simulink library "Simple_lib"  (R2018b)
settings: Solver=ode45  StartTime=0.0  StopTime=10.0  RelTol=1e-3  EnableMultiTasking=on
undefined symbols (not defined in the file or in its folder): Acceptance, beta, C, C_J, C_P, c_wall, dGain, DiscIntNeverNeededParam, Duplex, Electrical_lib, grab, h_fe, i, i3, K_T, Kman, KmanCE, mu_s, n_rev, R_arm, Simplex, systemTs, tau_0, TinIC, Ts, w_0, wallMass, Watch_lib
libraries: $bdroot x407, PlantUtilityBlockset_lib x30, peGeneralControl x22, simulink x11
(part 13 of 14)

== system Simple_lib/Driveline/Changan Transmission/Synchro2/Push_out ==
  InPot : Inport
  InFlow : Inport  Tag=NOFLUX  Port=2
  OutPot : Outport  Tag=NOFLUX
  tag scope: Push_outSynchro2TransmissionHYBPTPlantHybpt_test=global
  wires:
  InPot/1 -> OutPot/1  "pot"
  InFlow/1 -> [Push_outSynchro2TransmissionHYBPTPlantHybpt_test]  "flow"

== system Simple_lib/Driveline/Changan Transmission/Synchro2/Static Friction ==
  cap : Inport
  Dw : Inport  Port=2
  w : Inport  Port=3
  Tq : Inport  Port=4
  1/R2 : Gain  Gain=mu_s/2
  Abs : Abs
  Abs1 : Abs
  Abs2 : Abs
  Delay : Delay  DelayLength=1  InitialCondition=0
  Discrete-Time Integrator : DiscreteIntegrator  gainval=k_static  ExternalReset=level  SampleTime=Ts  ICPrevOutput=DiscIntNeverNeededParam  ICPrevScaledInput=DiscIntNeverNeededParam
  Logical Operator : Logic  Operator=OR  AllPortsSameDT=off  OutDataTypeStr=boolean
  Logical Operator1 : Logic  AllPortsSameDT=off  OutDataTypeStr=boolean
  Logical Operator2 : Logic  Operator=NOT  Inputs=1  AllPortsSameDT=off  OutDataTypeStr=boolean
  Relational Operator : RelationalOperator  OutDataTypeStr=boolean  RndMeth=Nearest
  Relational Operator1 : RelationalOperator  OutDataTypeStr=boolean  RndMeth=Nearest
  Saturation1 : Saturate  UpperLimit=inf  LowerLimit=0
  Sum2 : Sum  Inputs=-++
  big speed diff : Scope
  capacity : Scope
  oldtrans_exceeds_cap : Scope
  slipping : Scope
  Tq_stat : Outport
  wires:
  1/R2/1 -> Relational Operator/2
  Relational Operator/1 -> Logical Operator/1, big speed diff/1
  cap/1 -> capacity/1, Saturation1/1
  Logical Operator/1 -> slipping/1, Discrete-Time Integrator/2
  Discrete-Time Integrator/1 -> Tq_stat/1
  Abs/1 -> Relational Operator/1
  Abs2/1 -> Relational Operator1/1
  Saturation1/1 -> Relational Operator1/2
  Abs1/1 -> 1/R2/1
  Logical Operator1/1 -> oldtrans_exceeds_cap/1, Logical Operator/2
  Sum2/1 -> Abs1/1
  Tq/1 -> Abs2/1
  w/1 -> Sum2/2, Sum2/3
  Dw/1 -> Discrete-Time Integrator/1, Abs/1, Sum2/1
  Relational Operator1/1 -> Delay/1, Logical Operator1/1
  Delay/1 -> Logical Operator2/1
  Logical Operator2/1 -> Logical Operator1/2

== system Simple_lib/Driveline/Changan Transmission/Synchro3/Dynamic Friction ==
  Dw : Inport
  cap : Inport  Port=2
  Product : Product  RndMeth=Zero
  Saturation : Saturate  UpperLimit=inf  LowerLimit=0
  friction : Trigonometry  Operator=tanh
  grab : Gain  Gain=grab
  Tq_dyn : Outport
  wires:
  Dw/1 -> grab/1
  grab/1 -> friction/1
  friction/1 -> Product/2
  cap/1 -> Saturation/1
  Saturation/1 -> Product/1
  Product/1 -> Tq_dyn/1

== system Simple_lib/Driveline/Changan Transmission/Synchro3/Push_in ==
  InPot : Inport
  InFlow : Inport  Tag=NOFLUX  Port=2
  OutPot : Outport  Tag=NOFLUX
  tag scope: Push_inSynchro3TransmissionHYBPTPlantHybpt_test=global
  wires:
  InPot/1 -> OutPot/1  "pot"
  InFlow/1 -> [Push_inSynchro3TransmissionHYBPTPlantHybpt_test]  "flow"

== system Simple_lib/Driveline/Changan Transmission/Synchro3/Push_out ==
  InPot : Inport
  InFlow : Inport  Tag=NOFLUX  Port=2
  OutPot : Outport  Tag=NOFLUX
  tag scope: Push_outSynchro3TransmissionHYBPTPlantHybpt_test=global
  wires:
  InPot/1 -> OutPot/1  "pot"
  InFlow/1 -> [Push_outSynchro3TransmissionHYBPTPlantHybpt_test]  "flow"

== system Simple_lib/Driveline/Changan Transmission/Synchro3/Static Friction ==
  cap : Inport
  Dw : Inport  Port=2
  w : Inport  Port=3
  Tq : Inport  Port=4
  1/R2 : Gain  Gain=mu_s/2
  Abs : Abs
  Abs1 : Abs
  Abs2 : Abs
  Delay : Delay  DelayLength=1  InitialCondition=0
  Discrete-Time Integrator : DiscreteIntegrator  gainval=k_static  ExternalReset=level  SampleTime=Ts  ICPrevOutput=DiscIntNeverNeededParam  ICPrevScaledInput=DiscIntNeverNeededParam
  Logical Operator : Logic  Operator=OR  AllPortsSameDT=off  OutDataTypeStr=boolean
  Logical Operator1 : Logic  AllPortsSameDT=off  OutDataTypeStr=boolean
  Logical Operator2 : Logic  Operator=NOT  Inputs=1  AllPortsSameDT=off  OutDataTypeStr=boolean
  Relational Operator : RelationalOperator  OutDataTypeStr=boolean  RndMeth=Nearest
  Relational Operator1 : RelationalOperator  OutDataTypeStr=boolean  RndMeth=Nearest
  Saturation1 : Saturate  UpperLimit=inf  LowerLimit=0
  Sum2 : Sum  Inputs=-++
  big speed diff : Scope
  capacity : Scope
  oldtrans_exceeds_cap : Scope
  slipping : Scope
  Tq_stat : Outport
  wires:
  1/R2/1 -> Relational Operator/2
  Relational Operator/1 -> Logical Operator/1, big speed diff/1
  cap/1 -> capacity/1, Saturation1/1
  Logical Operator/1 -> slipping/1, Discrete-Time Integrator/2
  Discrete-Time Integrator/1 -> Tq_stat/1
  Abs/1 -> Relational Operator/1
  Abs2/1 -> Relational Operator1/1
  Saturation1/1 -> Relational Operator1/2
  Abs1/1 -> 1/R2/1
  Logical Operator1/1 -> oldtrans_exceeds_cap/1, Logical Operator/2
  Sum2/1 -> Abs1/1
  Tq/1 -> Abs2/1
  w/1 -> Sum2/2, Sum2/3
  Dw/1 -> Discrete-Time Integrator/1, Abs/1, Sum2/1
  Relational Operator1/1 -> Delay/1, Logical Operator1/1
  Delay/1 -> Logical Operator2/1
  Logical Operator2/1 -> Logical Operator1/2

== system Simple_lib/Driveline/Changan Transmission/Synchro4/Dynamic Friction ==
  Dw : Inport
  cap : Inport  Port=2
  Product : Product  RndMeth=Zero
  Saturation : Saturate  UpperLimit=inf  LowerLimit=0
  friction : Trigonometry  Operator=tanh
  grab : Gain  Gain=grab
  Tq_dyn : Outport
  wires:
  Dw/1 -> grab/1
  grab/1 -> friction/1
  friction/1 -> Product/2
  cap/1 -> Saturation/1
  Saturation/1 -> Product/1
  Product/1 -> Tq_dyn/1

== system Simple_lib/Driveline/Changan Transmission/Synchro4/Push_in ==
  InPot : Inport
  InFlow : Inport  Tag=NOFLUX  Port=2
  OutPot : Outport  Tag=NOFLUX
  tag scope: Push_inSynchro4TransmissionHYBPTPlantHybpt_test=global
  wires:
  InPot/1 -> OutPot/1  "pot"
  InFlow/1 -> [Push_inSynchro4TransmissionHYBPTPlantHybpt_test]  "flow"

== system Simple_lib/Driveline/Changan Transmission/Synchro4/Push_out ==
  InPot : Inport
  InFlow : Inport  Tag=NOFLUX  Port=2
  OutPot : Outport  Tag=NOFLUX
  tag scope: Push_outSynchro4TransmissionHYBPTPlantHybpt_test=global
  wires:
  InPot/1 -> OutPot/1  "pot"
  InFlow/1 -> [Push_outSynchro4TransmissionHYBPTPlantHybpt_test]  "flow"

== system Simple_lib/Driveline/Changan Transmission/Synchro4/Static Friction ==
  cap : Inport
  Dw : Inport  Port=2
  w : Inport  Port=3
  Tq : Inport  Port=4
  1/R2 : Gain  Gain=mu_s/2
  Abs : Abs
  Abs1 : Abs
  Abs2 : Abs
  Delay : Delay  DelayLength=1  InitialCondition=0
  Discrete-Time Integrator : DiscreteIntegrator  gainval=k_static  ExternalReset=level  SampleTime=Ts  ICPrevOutput=DiscIntNeverNeededParam  ICPrevScaledInput=DiscIntNeverNeededParam
  Logical Operator : Logic  Operator=OR  AllPortsSameDT=off  OutDataTypeStr=boolean
  Logical Operator1 : Logic  AllPortsSameDT=off  OutDataTypeStr=boolean
  Logical Operator2 : Logic  Operator=NOT  Inputs=1  AllPortsSameDT=off  OutDataTypeStr=boolean
  Relational Operator : RelationalOperator  OutDataTypeStr=boolean  RndMeth=Nearest
  Relational Operator1 : RelationalOperator  OutDataTypeStr=boolean  RndMeth=Nearest
  Saturation1 : Saturate  UpperLimit=inf  LowerLimit=0
  Sum2 : Sum  Inputs=-++
  big speed diff : Scope
  capacity : Scope
  oldtrans_exceeds_cap : Scope
  slipping : Scope
  Tq_stat : Outport
  wires:
  1/R2/1 -> Relational Operator/2
  Relational Operator/1 -> Logical Operator/1, big speed diff/1
  cap/1 -> capacity/1, Saturation1/1
  Logical Operator/1 -> slipping/1, Discrete-Time Integrator/2
  Discrete-Time Integrator/1 -> Tq_stat/1
  Abs/1 -> Relational Operator/1
  Abs2/1 -> Relational Operator1/1
  Saturation1/1 -> Relational Operator1/2
  Abs1/1 -> 1/R2/1
  Logical Operator1/1 -> oldtrans_exceeds_cap/1, Logical Operator/2
  Sum2/1 -> Abs1/1
  Tq/1 -> Abs2/1
  w/1 -> Sum2/2, Sum2/3
  Dw/1 -> Discrete-Time Integrator/1, Abs/1, Sum2/1
  Relational Operator1/1 -> Delay/1, Logical Operator1/1
  Delay/1 -> Logical Operator2/1
  Logical Operator2/1 -> Logical Operator1/2

== system Simple_lib/Driveline/Changan Transmission/Synchro5/Dynamic Friction ==
  Dw : Inport
  cap : Inport  Port=2
  Product : Product  RndMeth=Zero
  Saturation : Saturate  UpperLimit=inf  LowerLimit=0
  friction : Trigonometry  Operator=tanh
  grab : Gain  Gain=grab
  Tq_dyn : Outport
  wires:
  Dw/1 -> grab/1
  grab/1 -> friction/1
  friction/1 -> Product/2
  cap/1 -> Saturation/1
  Saturation/1 -> Product/1
  Product/1 -> Tq_dyn/1

== system Simple_lib/Driveline/Changan Transmission/Synchro5/Push_in ==
  InPot : Inport
  InFlow : Inport  Tag=NOFLUX  Port=2
  OutPot : Outport  Tag=NOFLUX
  tag scope: Push_inSynchro5TransmissionHYBPTPlantHybpt_test=global
  wires:
  InPot/1 -> OutPot/1  "pot"
  InFlow/1 -> [Push_inSynchro5TransmissionHYBPTPlantHybpt_test]  "flow"

== system Simple_lib/Driveline/Changan Transmission/Synchro5/Push_out ==
  InPot : Inport
  InFlow : Inport  Tag=NOFLUX  Port=2
  OutPot : Outport  Tag=NOFLUX
  tag scope: Push_outSynchro5TransmissionHYBPTPlantHybpt_test=global
  wires:
  InPot/1 -> OutPot/1  "pot"
  InFlow/1 -> [Push_outSynchro5TransmissionHYBPTPlantHybpt_test]  "flow"

== system Simple_lib/Driveline/Changan Transmission/Synchro5/Static Friction ==
  cap : Inport
  Dw : Inport  Port=2
  w : Inport  Port=3
  Tq : Inport  Port=4
  1/R2 : Gain  Gain=mu_s/2
  Abs : Abs
  Abs1 : Abs
  Abs2 : Abs
  Delay : Delay  DelayLength=1  InitialCondition=0
  Discrete-Time Integrator : DiscreteIntegrator  gainval=k_static  ExternalReset=level  SampleTime=Ts  ICPrevOutput=DiscIntNeverNeededParam  ICPrevScaledInput=DiscIntNeverNeededParam
  Logical Operator : Logic  Operator=OR  AllPortsSameDT=off  OutDataTypeStr=boolean
  Logical Operator1 : Logic  AllPortsSameDT=off  OutDataTypeStr=boolean
  Logical Operator2 : Logic  Operator=NOT  Inputs=1  AllPortsSameDT=off  OutDataTypeStr=boolean
  Relational Operator : RelationalOperator  OutDataTypeStr=boolean  RndMeth=Nearest
  Relational Operator1 : RelationalOperator  OutDataTypeStr=boolean  RndMeth=Nearest
  Saturation1 : Saturate  UpperLimit=inf  LowerLimit=0
  Sum2 : Sum  Inputs=-++
  big speed diff : Scope
  capacity : Scope
  oldtrans_exceeds_cap : Scope
  slipping : Scope
  Tq_stat : Outport
  wires:
  1/R2/1 -> Relational Operator/2
  Relational Operator/1 -> Logical Operator/1, big speed diff/1
  cap/1 -> capacity/1, Saturation1/1
  Logical Operator/1 -> slipping/1, Discrete-Time Integrator/2
  Discrete-Time Integrator/1 -> Tq_stat/1
  Abs/1 -> Relational Operator/1
  Abs2/1 -> Relational Operator1/1
  Saturation1/1 -> Relational Operator1/2
  Abs1/1 -> 1/R2/1
  Logical Operator1/1 -> oldtrans_exceeds_cap/1, Logical Operator/2
  Sum2/1 -> Abs1/1
  Tq/1 -> Abs2/1
  w/1 -> Sum2/2, Sum2/3
  Dw/1 -> Discrete-Time Integrator/1, Abs/1, Sum2/1
  Relational Operator1/1 -> Delay/1, Logical Operator1/1
  Delay/1 -> Logical Operator2/1
  Logical Operator2/1 -> Logical Operator1/2

== system Simple_lib/Driveline/Changan Transmission/Synchro6/Dynamic Friction ==
  Dw : Inport
  cap : Inport  Port=2
  Product : Product  RndMeth=Zero
  Saturation : Saturate  UpperLimit=inf  LowerLimit=0
  friction : Trigonometry  Operator=tanh
  grab : Gain  Gain=grab
  Tq_dyn : Outport
  wires:
  Dw/1 -> grab/1
  grab/1 -> friction/1
  friction/1 -> Product/2
  cap/1 -> Saturation/1
  Saturation/1 -> Product/1
  Product/1 -> Tq_dyn/1

== system Simple_lib/Driveline/Changan Transmission/Synchro6/Push_in ==
  InPot : Inport
  InFlow : Inport  Tag=NOFLUX  Port=2
  OutPot : Outport  Tag=NOFLUX
  tag scope: Push_inSynchro6TransmissionHYBPTPlantHybpt_test=global
  wires:
  InPot/1 -> OutPot/1  "pot"
  InFlow/1 -> [Push_inSynchro6TransmissionHYBPTPlantHybpt_test]  "flow"

== system Simple_lib/Driveline/Changan Transmission/Synchro6/Push_out ==
  InPot : Inport
  InFlow : Inport  Tag=NOFLUX  Port=2
  OutPot : Outport  Tag=NOFLUX
  tag scope: Push_outSynchro6TransmissionHYBPTPlantHybpt_test=global
  wires:
  InPot/1 -> OutPot/1  "pot"
  InFlow/1 -> [Push_outSynchro6TransmissionHYBPTPlantHybpt_test]  "flow"

== system Simple_lib/Driveline/Changan Transmission/Synchro6/Static Friction ==
  cap : Inport
  Dw : Inport  Port=2
  w : Inport  Port=3
  Tq : Inport  Port=4
  1/R2 : Gain  Gain=mu_s/2
  Abs : Abs
  Abs1 : Abs
  Abs2 : Abs
  Delay : Delay  DelayLength=1  InitialCondition=0
  Discrete-Time Integrator : DiscreteIntegrator  gainval=k_static  ExternalReset=level  SampleTime=Ts  ICPrevOutput=DiscIntNeverNeededParam  ICPrevScaledInput=DiscIntNeverNeededParam
  Logical Operator : Logic  Operator=OR  AllPortsSameDT=off  OutDataTypeStr=boolean
  Logical Operator1 : Logic  AllPortsSameDT=off  OutDataTypeStr=boolean
  Logical Operator2 : Logic  Operator=NOT  Inputs=1  AllPortsSameDT=off  OutDataTypeStr=boolean
  Relational Operator : RelationalOperator  OutDataTypeStr=boolean  RndMeth=Nearest
  Relational Operator1 : RelationalOperator  OutDataTypeStr=boolean  RndMeth=Nearest
  Saturation1 : Saturate  UpperLimit=inf  LowerLimit=0
  Sum2 : Sum  Inputs=-++
  big speed diff : Scope
  capacity : Scope
  oldtrans_exceeds_cap : Scope
  slipping : Scope
  Tq_stat : Outport
  wires:
  1/R2/1 -> Relational Operator/2
  Relational Operator/1 -> Logical Operator/1, big speed diff/1
  cap/1 -> capacity/1, Saturation1/1
  Logical Operator/1 -> slipping/1, Discrete-Time Integrator/2
  Discrete-Time Integrator/1 -> Tq_stat/1
  Abs/1 -> Relational Operator/1
  Abs2/1 -> Relational Operator1/1
  Saturation1/1 -> Relational Operator1/2
  Abs1/1 -> 1/R2/1
  Logical Operator1/1 -> oldtrans_exceeds_cap/1, Logical Operator/2
  Sum2/1 -> Abs1/1
  Tq/1 -> Abs2/1
  w/1 -> Sum2/2, Sum2/3
  Dw/1 -> Discrete-Time Integrator/1, Abs/1, Sum2/1
  Relational Operator1/1 -> Delay/1, Logical Operator1/1
  Delay/1 -> Logical Operator2/1
  Logical Operator2/1 -> Logical Operator1/2

== system Simple_lib/Driveline/diff_R/Carrier/Duplex ==
  InPot : Inport  Tag=NOFLUX
  FlowGain : Gain
  FlowSum : Sum  Inputs=2  SaturateOnIntegerOverflow=on  InputSameDT=on  OutDataTypeStr=Inherit: Same as first input
  OutPot : Outport
  OutFlow : Outport  Tag=NOFLUX  Port=2
  wires:
  FlowGain/1 -> OutFlow/1  "out_DuplexCarrierdiff_RBEVPlantBEV"
  InPot/1 -> OutPot/1  "DuplexCarrierdiff_RBEVPlantBEV"
  FlowSum/1 -> FlowGain/1
  [SimplexTransducerERADBEVPlantBEV] -> FlowSum/1
  [PushInertiaERADBEVPlantBEV] -> FlowSum/2

== system Simple_lib/Driveline/diff_R/Carrier/Simplex ==
  InPot : Inport
  InFlow : Inport  Tag=NOFLUX  Port=2
  OutPot : Outport  Tag=NOFLUX
  tag scope: SimplexCarrierdiff_RBEVPlantBEV=global
  wires:
  InPot/1 -> OutPot/1  "SimplexCarrierdiff_RBEVPlantBEV"
  InFlow/1 -> [SimplexCarrierdiff_RBEVPlantBEV]  "out_SimplexCarrierdiff_RBEVPlantBEV"

== system Simple_lib/Driveline/diff_R/Carrier/Simplex1 ==
  InPot : Inport
  InFlow : Inport  Tag=NOFLUX  Port=2
  OutPot : Outport  Tag=NOFLUX
  tag scope: Simplex1Carrierdiff_RBEVPlantBEV=global
  wires:
  InPot/1 -> OutPot/1  "Simplex1Carrierdiff_RBEVPlantBEV"
  InFlow/1 -> [Simplex1Carrierdiff_RBEVPlantBEV]  "out_Simplex1Carrierdiff_RBEVPlantBEV"

== system Simple_lib/Driveline/diff_R/GearPair /Pull ==
  InPot : Inport  Tag=NOFLUX
  FlowGain : Gain
  OutPot : Outport
  OutFlow : Outport  Tag=NOFLUX  Port=2
  wires:
  FlowGain/1 -> OutFlow/1  "out_PullGearPairdiff_RBEVPlantBEV"
  InPot/1 -> OutPot/1  "PullGearPairdiff_RBEVPlantBEV"
  [SimplexCarrierdiff_RBEVPlantBEV] -> FlowGain/1

== system Simple_lib/Driveline/diff_R/GearPair /Push ==
  InPot : Inport
  InFlow : Inport  Tag=NOFLUX  Port=2
  OutPot : Outport  Tag=NOFLUX
  tag scope: PushGearPairdiff_RBEVPlantBEV=global
  wires:
  InPot/1 -> OutPot/1  "PushGearPairdiff_RBEVPlantBEV"
  InFlow/1 -> [PushGearPairdiff_RBEVPlantBEV]  "out_PushGearPairdiff_RBEVPlantBEV"

== system Simple_lib/Driveline/diff_R/GearPair 1/Pull ==
  InPot : Inport  Tag=NOFLUX
  FlowGain : Gain
  OutPot : Outport
  OutFlow : Outport  Tag=NOFLUX  Port=2
  wires:
  FlowGain/1 -> OutFlow/1  "out_PullGearPair1diff_RBEVPlantBEV"
  InPot/1 -> OutPot/1  "PullGearPair1diff_RBEVPlantBEV"
  [Simplex1Carrierdiff_RBEVPlantBEV] -> FlowGain/1

== system Simple_lib/Driveline/diff_R/GearPair 1/Push ==
  InPot : Inport
  InFlow : Inport  Tag=NOFLUX  Port=2
  OutPot : Outport  Tag=NOFLUX
  tag scope: PushGearPair1diff_RBEVPlantBEV=global
  wires:
  InPot/1 -> OutPot/1  "PushGearPair1diff_RBEVPlantBEV"
  InFlow/1 -> [PushGearPair1diff_RBEVPlantBEV]  "out_PushGearPair1diff_RBEVPlantBEV"

== system Simple_lib/Electrical/B2/C/Duplex ==
  potential : Inport  Tag=NOFLUX
  Display1 : Display
  duplexFluxSum : Sum  Inputs=2  SaturateOnIntegerOverflow=on  InputSameDT=on  OutDataTypeStr=Inherit: Same as first input
  fDuplexR1Duplicity1 : Scope
  pDuplexR1Duplicity1 : Scope
  potDisplay : Display
  duplex : Outport
  flow : Outport  Tag=NOFLUX  Port=2
  wires:
  potential/1 -> pDuplexR1Duplicity1/1, potDisplay/1, duplex/1
  duplexFluxSum/1 -> Display1/1, fDuplexR1Duplicity1/1, flow/1
  [duplexSimplexR0B1Duplicity1] -> duplexFluxSum/1
  [duplexSimplex1LB1Duplicity1] -> duplexFluxSum/2

== system Simple_lib/Electrical/B2/E/Duplex ==
  potential : Inport  Tag=NOFLUX
  Display1 : Display
  duplexFluxSum : Gain  SaturateOnIntegerOverflow=on  OutDataTypeStr=Inherit: Same as input  ParamDataTypeStr=Inherit: Same as input
  fDuplexR1Duplicity1 : Scope
  pDuplexR1Duplicity1 : Scope
  potDisplay : Display
  duplex : Outport
  flow : Outport  Tag=NOFLUX  Port=2
  wires:
  potential/1 -> pDuplexR1Duplicity1/1, potDisplay/1, duplex/1
  duplexFluxSum/1 -> Display1/1, fDuplexR1Duplicity1/1, flow/1
  [duplexSimplexLB1Duplicity1] -> duplexFluxSum/1

== system Simple_lib/Electrical/B2/E/Simplex ==
  duplex : Inport
  In2 : Inport  Tag=NOFLUX  Port=2
  fSimplexR1Duplicity1 : Scope
  flowDisplay : Display
  fluxduplexGain : Gain  SaturateOnIntegerOverflow=on  OutDataTypeStr=Inherit: Same as input  ParamDataTypeStr=Inherit: Same as input
  pSimplexR1Duplicity1 : Scope
  potDisplay : Display
  simplex : Outport  Tag=NOFLUX
  tag scope: duplexSimplexEB1Duplicity1=global
  wires:
  In2/1 -> fSimplexR1Duplicity1/1, fluxduplexGain/1, flowDisplay/1
  fluxduplexGain/1 -> [duplexSimplexEB1Duplicity1]
  duplex/1 -> potDisplay/1, pSimplexR1Duplicity1/1, simplex/1

== system Simple_lib/Electrical/B2/L/Simplex ==
  duplex : Inport
  In2 : Inport  Tag=NOFLUX  Port=2
  fSimplexR1Duplicity1 : Scope
  flowDisplay : Display
  fluxduplexGain : Gain  SaturateOnIntegerOverflow=on  OutDataTypeStr=Inherit: Same as input  ParamDataTypeStr=Inherit: Same as input
  pSimplexR1Duplicity1 : Scope
  potDisplay : Display
  simplex : Outport  Tag=NOFLUX
  tag scope: duplexSimplexLB1Duplicity1=global
  wires:
  In2/1 -> fSimplexR1Duplicity1/1, fluxduplexGain/1, flowDisplay/1
  fluxduplexGain/1 -> [duplexSimplexLB1Duplicity1]
  duplex/1 -> potDisplay/1, pSimplexR1Duplicity1/1, simplex/1

== system Simple_lib/Electrical/B2/L/Simplex1 ==
  duplex : Inport
  In2 : Inport  Tag=NOFLUX  Port=2
  fSimplexR1Duplicity1Simplex1LB1Duplicity1 : Scope
  flowDisplay : Display
  fluxduplexGain : Gain  SaturateOnIntegerOverflow=on  OutDataTypeStr=Inherit: Same as input  ParamDataTypeStr=Inherit: Same as input
  pSimplexR1Duplicity1Simplex1LB1Duplicity1 : Scope
  potDisplay : Display
  simplex : Outport  Tag=NOFLUX
  tag scope: duplexSimplex1LB1Duplicity1=global
  wires:
  In2/1 -> fSimplexR1Duplicity1Simplex1LB1Duplicity1/1, fluxduplexGain/1, flowDisplay/1
  fluxduplexGain/1 -> [duplexSimplex1LB1Duplicity1]
  duplex/1 -> potDisplay/1, pSimplexR1Duplicity1Simplex1LB1Duplicity1/1, simplex/1

== system Simple_lib/Electrical/B2/R0/Duplex ==
  potential : Inport  Tag=NOFLUX
  Display1 : Display
  duplexFluxSum : Gain  SaturateOnIntegerOverflow=on  OutDataTypeStr=Inherit: Same as input  ParamDataTypeStr=Inherit: Same as input
  fDuplexR1Duplicity1 : Scope
  pDuplexR1Duplicity1 : Scope
  potDisplay : Display
  duplex : Outport
  flow : Outport  Tag=NOFLUX  Port=2
  wires:
  potential/1 -> pDuplexR1Duplicity1/1, potDisplay/1, duplex/1
  duplexFluxSum/1 -> Display1/1, fDuplexR1Duplicity1/1, flow/1
  [duplexSimplexR1Duplicity1] -> duplexFluxSum/1

== system Simple_lib/Electrical/B2/R0/Simplex ==
  duplex : Inport
  In2 : Inport  Tag=NOFLUX  Port=2
  fSimplexR1Duplicity1 : Scope
  flowDisplay : Display
  fluxduplexGain : Gain  SaturateOnIntegerOverflow=on  OutDataTypeStr=Inherit: Same as input  ParamDataTypeStr=Inherit: Same as input
  pSimplexR1Duplicity1 : Scope
  potDisplay : Display
  simplex : Outport  Tag=NOFLUX
  tag scope: duplexSimplexR0B1Duplicity1=global
  wires:
  In2/1 -> fSimplexR1Duplicity1/1, fluxduplexGain/1, flowDisplay/1
  fluxduplexGain/1 -> [duplexSimplexR0B1Duplicity1]
  duplex/1 -> potDisplay/1, pSimplexR1Duplicity1/1, simplex/1

== system Simple_lib/Electrical/SimplestEMachine/Inertia/Push ==
  InPot : Inport
  InFlow : Inport  Tag=NOFLUX  Port=2
  OutPot : Outport  Tag=NOFLUX
  tag scope: PushInertiaEFADBEVPlantBEV=global
  wires:
  InPot/1 -> OutPot/1  "PushInertiaEFADBEVPlantBEV"
  InFlow/1 -> [PushInertiaEFADBEVPlantBEV]  "out_PushInertiaEFADBEVPlantBEV"

== system Simple_lib/Electrical/SimplestEMachine/Transducer/Duplex ==
  InPot : Inport  Tag=NOFLUX
  FlowGain : Gain
  OutPot : Outport
  OutFlow : Outport  Tag=NOFLUX  Port=2
  wires:
  [SimplexInverter_FBEVPlantBEV] -> FlowGain/1
  InPot/1 -> OutPot/1  "DuplexTransducerEFADBEVPlantBEV"
  FlowGain/1 -> OutFlow/1  "out_DuplexTransducerEFADBEVPlantBEV"

== system Simple_lib/Electrical/SimplestEMachine/Transducer/Simplex ==
  InPot : Inport
  InFlow : Inport  Tag=NOFLUX  Port=2
  OutPot : Outport  Tag=NOFLUX
  tag scope: SimplexTransducerEFADBEVPlantBEV=global
  wires:
  InFlow/1 -> [SimplexTransducerEFADBEVPlantBEV]  "out_SimplexTransducerEFADBEVPlantBEV"
  InPot/1 -> OutPot/1  "SimplexTransducerEFADBEVPlantBEV"

== system Simple_lib/Electrical/Windings/IM/Duplex ==
  InPot : Inport  Tag=NOFLUX
  FlowDisplay : Display
  FlowGain : Gain
  Flow_DuplexIMWindingsMk4v3Inverter_test0 : Scope
      settings: Tag=Flow
  PotDisplay : Display
  Pot_DuplexIMWindingsMk4v3Inverter_test0 : Scope
      settings: Tag=Pot
  Rate Transition : RateTransition  OutPortSampleTimeMultiple=nT  OutPortSampleTime=Ts
  OutPot : Outport
  OutFlow : Outport  Tag=NOFLUX  Port=2
  wires:
  Rate Transition/1 -> OutPot/1
  InPot/1 -> Rate Transition/1, PotDisplay/1, Pot_DuplexIMWindingsMk4v3Inverter_test0/1
  FlowGain/1 -> OutFlow/1, FlowDisplay/1, Flow_DuplexIMWindingsMk4v3Inverter_test0/1
  [SimplexL1WindingsMk4v3Inverter_test0] -> FlowGain/1

== system Simple_lib/Electrical/Windings/IM/Simplex ==
  InPot : Inport
  InFlow : Inport  Tag=NOFLUX  Port=2
  FlowDisplay : Display
  Flow_SimplexIMWindingsMk4v3Inverter_test0 : Scope
      settings: Tag=Flow
  PotDisplay : Display
  Pot_SimplexIMWindingsMk4v3Inverter_test0 : Scope
      settings: Tag=Pot
  Rate Transition : RateTransition  OutPortSampleTimeMultiple=Ts  OutPortSampleTime=Ts
  OutPot : Outport  Tag=NOFLUX
  tag scope: SimplexIMWindingsMk4v3Inverter_test0=global
  wires:
  InPot/1 -> Rate Transition/1
  InFlow/1 -> Flow_SimplexIMWindingsMk4v3Inverter_test0/1, FlowDisplay/1, [SimplexIMWindingsMk4v3Inverter_test0]
  Rate Transition/1 -> OutPot/1, Pot_SimplexIMWindingsMk4v3Inverter_test0/1, PotDisplay/1

== system Simple_lib/Electrical/Windings/IM1/Duplex ==
  InPot : Inport  Tag=NOFLUX
  FlowDisplay : Display
  FlowGain : Gain
  Flow_DuplexIM1WindingsMk4v3Inverter_test0 : Scope
      settings: Tag=Flow
  PotDisplay : Display
  Pot_DuplexIM1WindingsMk4v3Inverter_test0 : Scope
      settings: Tag=Pot
  Rate Transition : RateTransition  OutPortSampleTimeMultiple=nT  OutPortSampleTime=Ts
  OutPot : Outport
  OutFlow : Outport  Tag=NOFLUX  Port=2
  wires:
  Rate Transition/1 -> OutPot/1
  InPot/1 -> Rate Transition/1, PotDisplay/1, Pot_DuplexIM1WindingsMk4v3Inverter_test0/1
  FlowGain/1 -> OutFlow/1, Flow_DuplexIM1WindingsMk4v3Inverter_test0/1, FlowDisplay/1
  [SimplexL2WindingsMk4v3Inverter_test0] -> FlowGain/1

== system Simple_lib/Electrical/Windings/IM1/Simplex ==
  InPot : Inport
  InFlow : Inport  Tag=NOFLUX  Port=2
  FlowDisplay : Display
  Flow_SimplexIM1WindingsMk4v3Inverter_test0 : Scope
      settings: Tag=Flow
  PotDisplay : Display
  Pot_SimplexIM1WindingsMk4v3Inverter_test0 : Scope
      settings: Tag=Pot
  Rate Transition : RateTransition  OutPortSampleTimeMultiple=Ts  OutPortSampleTime=Ts
  OutPot : Outport  Tag=NOFLUX
  tag scope: SimplexIM1WindingsMk4v3Inverter_test0=global
  wires:
  InPot/1 -> Rate Transition/1
  InFlow/1 -> Flow_SimplexIM1WindingsMk4v3Inverter_test0/1, FlowDisplay/1, [SimplexIM1WindingsMk4v3Inverter_test0]
  Rate Transition/1 -> OutPot/1, Pot_SimplexIM1WindingsMk4v3Inverter_test0/1, PotDisplay/1

== system Simple_lib/Electrical/Windings/IM2/Duplex ==
  InPot : Inport  Tag=NOFLUX
  FlowDisplay : Display
  FlowGain : Gain
  Flow_DuplexIM2WindingsMk4v3Inverter_test0 : Scope
      settings: Tag=Flow
  PotDisplay : Display
  Pot_DuplexIM2WindingsMk4v3Inverter_test0 : Scope
      settings: Tag=Pot
  Rate Transition : RateTransition  OutPortSampleTimeMultiple=nT  OutPortSampleTime=Ts
  OutPot : Outport
  OutFlow : Outport  Tag=NOFLUX  Port=2
  wires:
  Rate Transition/1 -> OutPot/1
  InPot/1 -> Rate Transition/1, PotDisplay/1, Pot_DuplexIM2WindingsMk4v3Inverter_test0/1
  FlowGain/1 -> OutFlow/1, Flow_DuplexIM2WindingsMk4v3Inverter_test0/1, FlowDisplay/1
  [SimplexL3WindingsMk4v3Inverter_test0] -> FlowGain/1

== system Simple_lib/Electrical/Windings/IM2/Simplex ==
  InPot : Inport
  InFlow : Inport  Tag=NOFLUX  Port=2
  FlowDisplay : Display
  Flow_SimplexIM2WindingsMk4v3Inverter_test0 : Scope
      settings: Tag=Flow
  PotDisplay : Display
  Pot_SimplexIM2WindingsMk4v3Inverter_test0 : Scope
      settings: Tag=Pot
  Rate Transition : RateTransition  OutPortSampleTimeMultiple=Ts  OutPortSampleTime=Ts
  OutPot : Outport  Tag=NOFLUX
  tag scope: SimplexIM2WindingsMk4v3Inverter_test0=global
  wires:
  InPot/1 -> Rate Transition/1
  InFlow/1 -> Flow_SimplexIM2WindingsMk4v3Inverter_test0/1, FlowDisplay/1, [SimplexIM2WindingsMk4v3Inverter_test0]
  Rate Transition/1 -> OutPot/1, Pot_SimplexIM2WindingsMk4v3Inverter_test0/1, PotDisplay/1

== system Simple_lib/Electrical/Windings/L1/Simplex ==
  InPot : Inport
  InFlow : Inport  Tag=NOFLUX  Port=2
  FlowDisplay : Display
  Flow_SimplexL1WindingsMk4v3Inverter_test0 : Scope
      settings: Tag=Flow
  PotDisplay : Display
  Pot_SimplexL1WindingsMk4v3Inverter_test0 : Scope
      settings: Tag=Pot
  Rate Transition : RateTransition  OutPortSampleTimeMultiple=Ts  OutPortSampleTime=Ts
  OutPot : Outport  Tag=NOFLUX
  tag scope: SimplexL1WindingsMk4v3Inverter_test0=global
  wires:
  InPot/1 -> Rate Transition/1
  InFlow/1 -> Flow_SimplexL1WindingsMk4v3Inverter_test0/1, FlowDisplay/1, [SimplexL1WindingsMk4v3Inverter_test0]
  Rate Transition/1 -> OutPot/1, Pot_SimplexL1WindingsMk4v3Inverter_test0/1, PotDisplay/1

== system Simple_lib/Electrical/Windings/L1/Simplex1 ==
  InPot : Inport
  InFlow : Inport  Tag=NOFLUX  Port=2
  FlowDisplay : Display
  Flow_Simplex1L1WindingsMk4v3Inverter_test0 : Scope
      settings: Tag=Flow
  PotDisplay : Display
  Pot_Simplex1L1WindingsMk4v3Inverter_test0 : Scope
      settings: Tag=Pot
  Rate Transition : RateTransition  OutPortSampleTimeMultiple=Ts  OutPortSampleTime=Ts
  OutPot : Outport  Tag=NOFLUX
  tag scope: Simplex1L1WindingsMk4v3Inverter_test0=global
  wires:
  InPot/1 -> Rate Transition/1
  InFlow/1 -> Flow_Simplex1L1WindingsMk4v3Inverter_test0/1, FlowDisplay/1, [Simplex1L1WindingsMk4v3Inverter_test0]
  Rate Transition/1 -> OutPot/1, Pot_Simplex1L1WindingsMk4v3Inverter_test0/1, PotDisplay/1

== system Simple_lib/Electrical/Windings/L2/Simplex ==
  InPot : Inport
  InFlow : Inport  Tag=NOFLUX  Port=2
  FlowDisplay : Display
  Flow_SimplexL2WindingsMk4v3Inverter_test0 : Scope
      settings: Tag=Flow
  PotDisplay : Display
  Pot_SimplexL2WindingsMk4v3Inverter_test0 : Scope
      settings: Tag=Pot
  Rate Transition : RateTransition  OutPortSampleTimeMultiple=Ts  OutPortSampleTime=Ts
  OutPot : Outport  Tag=NOFLUX
  tag scope: SimplexL2WindingsMk4v3Inverter_test0=global
  wires:
  InPot/1 -> Rate Transition/1
  InFlow/1 -> Flow_SimplexL2WindingsMk4v3Inverter_test0/1, FlowDisplay/1, [SimplexL2WindingsMk4v3Inverter_test0]
  Rate Transition/1 -> OutPot/1, Pot_SimplexL2WindingsMk4v3Inverter_test0/1, PotDisplay/1

== system Simple_lib/Electrical/Windings/L2/Simplex1 ==
  InPot : Inport
  InFlow : Inport  Tag=NOFLUX  Port=2
  FlowDisplay : Display
  Flow_Simplex1L2WindingsMk4v3Inverter_test0 : Scope
      settings: Tag=Flow
  PotDisplay : Display
  Pot_Simplex1L2WindingsMk4v3Inverter_test0 : Scope
      settings: Tag=Pot
  Rate Transition : RateTransition  OutPortSampleTimeMultiple=Ts  OutPortSampleTime=Ts
  OutPot : Outport  Tag=NOFLUX
  tag scope: Simplex1L2WindingsMk4v3Inverter_test0=global
  wires:
  InPot/1 -> Rate Transition/1
  InFlow/1 -> Flow_Simplex1L2WindingsMk4v3Inverter_test0/1, FlowDisplay/1, [Simplex1L2WindingsMk4v3Inverter_test0]
  Rate Transition/1 -> OutPot/1, Pot_Simplex1L2WindingsMk4v3Inverter_test0/1, PotDisplay/1

== system Simple_lib/Electrical/Windings/L3/Simplex ==
  InPot : Inport
  InFlow : Inport  Tag=NOFLUX  Port=2
  FlowDisplay : Display
  Flow_SimplexL3WindingsMk4v3Inverter_test0 : Scope
      settings: Tag=Flow
  PotDisplay : Display
  Pot_SimplexL3WindingsMk4v3Inverter_test0 : Scope
      settings: Tag=Pot
  Rate Transition : RateTransition  OutPortSampleTimeMultiple=Ts  OutPortSampleTime=Ts
  OutPot : Outport  Tag=NOFLUX
  tag scope: SimplexL3WindingsMk4v3Inverter_test0=global
  wires:
  InPot/1 -> Rate Transition/1
  InFlow/1 -> Flow_SimplexL3WindingsMk4v3Inverter_test0/1, FlowDisplay/1, [SimplexL3WindingsMk4v3Inverter_test0]
  Rate Transition/1 -> OutPot/1, Pot_SimplexL3WindingsMk4v3Inverter_test0/1, PotDisplay/1

== system Simple_lib/Electrical/Windings/L3/Simplex1 ==
  InPot : Inport
  InFlow : Inport  Tag=NOFLUX  Port=2
  FlowDisplay : Display
  Flow_Simplex1L3WindingsMk4v3Inverter_test0 : Scope
      settings: Tag=Flow
  PotDisplay : Display
  Pot_Simplex1L3WindingsMk4v3Inverter_test0 : Scope
      settings: Tag=Pot
  Rate Transition : RateTransition  OutPortSampleTimeMultiple=Ts  OutPortSampleTime=Ts
  OutPot : Outport  Tag=NOFLUX
  tag scope: Simplex1L3WindingsMk4v3Inverter_test0=global
  wires:
  InPot/1 -> Rate Transition/1
  InFlow/1 -> Flow_Simplex1L3WindingsMk4v3Inverter_test0/1, FlowDisplay/1, [Simplex1L3WindingsMk4v3Inverter_test0]
  Rate Transition/1 -> OutPot/1, Pot_Simplex1L3WindingsMk4v3Inverter_test0/1, PotDisplay/1

== system Simple_lib/Electrical/Windings/R/Duplex ==
  InPot : Inport  Tag=NOFLUX
  FlowDisplay : Display
  FlowGain : Gain
  Flow_DuplexRWindingsMk4v3Inverter_test0 : Scope
      settings: Tag=Flow
  PotDisplay : Display
  Pot_DuplexRWindingsMk4v3Inverter_test0 : Scope
      settings: Tag=Pot
  Rate Transition : RateTransition  OutPortSampleTimeMultiple=nT  OutPortSampleTime=Ts
  OutPot : Outport
  OutFlow : Outport  Tag=NOFLUX  Port=2
  wires:
  Rate Transition/1 -> OutPot/1
  InPot/1 -> Rate Transition/1, PotDisplay/1, Pot_DuplexRWindingsMk4v3Inverter_test0/1
  FlowGain/1 -> OutFlow/1, Flow_DuplexRWindingsMk4v3Inverter_test0/1, FlowDisplay/1
  [SimplexIMWindingsMk4v3Inverter_test0] -> FlowGain/1

== system Simple_lib/Electrical/Windings/R/Simplex ==
  InPot : Inport
  InFlow : Inport  Tag=NOFLUX  Port=2
  FlowDisplay : Display
  Flow_SimplexRWindingsMk4v3Inverter_test0 : Scope
      settings: Tag=Flow
  PotDisplay : Display
  Pot_SimplexRWindingsMk4v3Inverter_test0 : Scope
      settings: Tag=Pot
  Rate Transition : RateTransition  OutPortSampleTimeMultiple=Ts  OutPortSampleTime=Ts
  OutPot : Outport  Tag=NOFLUX
  tag scope: SimplexRWindingsMk4v3Inverter_test0=global
  wires:
  InPot/1 -> Rate Transition/1
  InFlow/1 -> Flow_SimplexRWindingsMk4v3Inverter_test0/1, FlowDisplay/1, [SimplexRWindingsMk4v3Inverter_test0]
  Rate Transition/1 -> OutPot/1, Pot_SimplexRWindingsMk4v3Inverter_test0/1, PotDisplay/1

== system Simple_lib/Electrical/Windings/R1/Duplex ==
  InPot : Inport  Tag=NOFLUX
  FlowDisplay : Display
  FlowGain : Gain
  Flow_DuplexR1WindingsMk4v3Inverter_test0 : Scope
      settings: Tag=Flow
  PotDisplay : Display
  Pot_DuplexR1WindingsMk4v3Inverter_test0 : Scope
      settings: Tag=Pot
  Rate Transition : RateTransition  OutPortSampleTimeMultiple=nT  OutPortSampleTime=Ts
  OutPot : Outport
  OutFlow : Outport  Tag=NOFLUX  Port=2
  wires:
  Rate Transition/1 -> OutPot/1
  InPot/1 -> Rate Transition/1, PotDisplay/1, Pot_DuplexR1WindingsMk4v3Inverter_test0/1
  FlowGain/1 -> OutFlow/1, Flow_DuplexR1WindingsMk4v3Inverter_test0/1, FlowDisplay/1
  [SimplexIM1WindingsMk4v3Inverter_test0] -> FlowGain/1

== system Simple_lib/Electrical/Windings/R1/Simplex ==
  InPot : Inport
  InFlow : Inport  Tag=NOFLUX  Port=2
  FlowDisplay : Display
  Flow_SimplexR1WindingsMk4v3Inverter_test0 : Scope
      settings: Tag=Flow
  PotDisplay : Display
  Pot_SimplexR1WindingsMk4v3Inverter_test0 : Scope
      settings: Tag=Pot
  Rate Transition : RateTransition  OutPortSampleTimeMultiple=Ts  OutPortSampleTime=Ts
  OutPot : Outport  Tag=NOFLUX
  tag scope: SimplexR1WindingsMk4v3Inverter_test0=global
  wires:
  InPot/1 -> Rate Transition/1
  InFlow/1 -> Flow_SimplexR1WindingsMk4v3Inverter_test0/1, FlowDisplay/1, [SimplexR1WindingsMk4v3Inverter_test0]
  Rate Transition/1 -> OutPot/1, Pot_SimplexR1WindingsMk4v3Inverter_test0/1, PotDisplay/1

== system Simple_lib/Electrical/Windings/R2/Duplex ==
  InPot : Inport  Tag=NOFLUX
  FlowDisplay : Display
  FlowGain : Gain
  Flow_DuplexR2WindingsMk4v3Inverter_test0 : Scope
      settings: Tag=Flow
  PotDisplay : Display
  Pot_DuplexR2WindingsMk4v3Inverter_test0 : Scope
      settings: Tag=Pot
  Rate Transition : RateTransition  OutPortSampleTimeMultiple=nT  OutPortSampleTime=Ts
  OutPot : Outport
  OutFlow : Outport  Tag=NOFLUX  Port=2
  wires:
  Rate Transition/1 -> OutPot/1
  InPot/1 -> Rate Transition/1, PotDisplay/1, Pot_DuplexR2WindingsMk4v3Inverter_test0/1
  FlowGain/1 -> OutFlow/1, Flow_DuplexR2WindingsMk4v3Inverter_test0/1, FlowDisplay/1
  [SimplexIM2WindingsMk4v3Inverter_test0] -> FlowGain/1

== system Simple_lib/Electrical/Windings/R2/Simplex ==
  InPot : Inport
  InFlow : Inport  Tag=NOFLUX  Port=2
  FlowDisplay : Display
  Flow_SimplexR2WindingsMk4v3Inverter_test0 : Scope
      settings: Tag=Flow
  PotDisplay : Display
  Pot_SimplexR2WindingsMk4v3Inverter_test0 : Scope
      settings: Tag=Pot
  Rate Transition : RateTransition  OutPortSampleTimeMultiple=Ts  OutPortSampleTime=Ts
  OutPot : Outport  Tag=NOFLUX
  tag scope: SimplexR2WindingsMk4v3Inverter_test0=global
  wires:
  InPot/1 -> Rate Transition/1
  InFlow/1 -> Flow_SimplexR2WindingsMk4v3Inverter_test0/1, FlowDisplay/1, [SimplexR2WindingsMk4v3Inverter_test0]
  Rate Transition/1 -> OutPot/1, Pot_SimplexR2WindingsMk4v3Inverter_test0/1, PotDisplay/1

== system Simple_lib/Hydraulic/ Heat Exchanger/Linear Heat Pipe/Pull ==
  InPot : Inport  Tag=NOFLUX
  FlowDisplay : Display
  FlowGain : Gain
  Flow_PullLinearHeatPipeHeatExchangerFessSchematicSimulinkThermalFlui : Scope
      settings: Tag=Flow
  PotDisplay : Display
  Pot_PullLinearHeatPipeHeatExchangerFessSchematicSimulinkThermalFlui : Scope
      settings: Tag=Pot
  Rate Transition : RateTransition  OutPortSampleTimeMultiple=nT  OutPortSampleTime=Ts
  OutPot : Outport
  OutFlow : Outport  Tag=NOFLUX  Port=2
  wires:
  FlowGain/1 -> FlowDisplay/1, Flow_PullLinearHeatPipeHeatExchangerFessSchematicSimulinkThermalFlui/1, OutFlow/1
  InPot/1 -> Pot_PullLinearHeatPipeHeatExchangerFessSchematicSimulinkThermalFlui/1, PotDisplay/1, Rate Transition/1
  Rate Transition/1 -> OutPot/1

== system Simple_lib/Hydraulic/ Heat Exchanger/Linear Heat Pipe/Push ==
  InPot : Inport
  InFlow : Inport  Tag=NOFLUX  Port=2
  FlowDisplay : Display
  Flow_PushLinearHeatPipeHeatExchangerFessSchematicSimulinkThermalFlui : Scope
      settings: Tag=Flow
  PotDisplay : Display
  Pot_PushLinearHeatPipeHeatExchangerFessSchematicSimulinkThermalFlui : Scope
      settings: Tag=Pot
  Rate Transition : RateTransition  OutPortSampleTimeMultiple=Ts  OutPortSampleTime=Ts
  OutPot : Outport  Tag=NOFLUX
  tag scope: PushLinearHeatPipeHeatExchangerFessSchematicSimulinkThermalFlui=global
  wires:
  InPot/1 -> Rate Transition/1
  InFlow/1 -> Flow_PushLinearHeatPipeHeatExchangerFessSchematicSimulinkThermalFlui/1, FlowDisplay/1, [PushLinearHeatPipeHeatExchangerFessSchematicSimulinkThermalFlui]
  Rate Transition/1 -> OutPot/1, Pot_PushLinearHeatPipeHeatExchangerFessSchematicSimulinkThermalFlui/1, PotDisplay/1

== system Simple_lib/Hydraulic/ Heat Exchanger/Linear Heat Pipe1/Pull ==
  InPot : Inport  Tag=NOFLUX
  FlowDisplay : Display
  FlowGain : Gain
  Flow_PullLinearHeatPipe1HeatExchangerFessSchematicSimulinkThermalFlu : Scope
      settings: Tag=Flow
  PotDisplay : Display
  Pot_PullLinearHeatPipe1HeatExchangerFessSchematicSimulinkThermalFlu : Scope
      settings: Tag=Pot
  Rate Transition : RateTransition  OutPortSampleTimeMultiple=nT  OutPortSampleTime=Ts
  OutPot : Outport
  OutFlow : Outport  Tag=NOFLUX  Port=2
  wires:
  FlowGain/1 -> FlowDisplay/1, Flow_PullLinearHeatPipe1HeatExchangerFessSchematicSimulinkThermalFlu/1, OutFlow/1
  InPot/1 -> Pot_PullLinearHeatPipe1HeatExchangerFessSchematicSimulinkThermalFlu/1, PotDisplay/1, Rate Transition/1
  Rate Transition/1 -> OutPot/1

== system Simple_lib/Hydraulic/ Heat Exchanger/Linear Heat Pipe1/Push ==
  InPot : Inport
  InFlow : Inport  Tag=NOFLUX  Port=2
  FlowDisplay : Display
  Flow_PushLinearHeatPipe1HeatExchangerFessSchematicSimulinkThermalFlu : Scope
      settings: Tag=Flow
  PotDisplay : Display
  Pot_PushLinearHeatPipe1HeatExchangerFessSchematicSimulinkThermalFlu : Scope
      settings: Tag=Pot
  Rate Transition : RateTransition  OutPortSampleTimeMultiple=Ts  OutPortSampleTime=Ts
  OutPot : Outport  Tag=NOFLUX
  tag scope: PushLinearHeatPipe1HeatExchangerFessSchematicSimulinkThermalFlu=global
  wires:
  InPot/1 -> Rate Transition/1
  InFlow/1 -> Flow_PushLinearHeatPipe1HeatExchangerFessSchematicSimulinkThermalFlu/1, FlowDisplay/1, [PushLinearHeatPipe1HeatExchangerFessSchematicSimulinkThermalFlu]
  Rate Transition/1 -> OutPot/1, Pot_PushLinearHeatPipe1HeatExchangerFessSchematicSimulinkThermalFlu/1, PotDisplay/1

== system Simple_lib/Hydraulic/Heat Sink/Linear Heat Pipe1/Pull ==
  InPot : Inport  Tag=NOFLUX
  FlowDisplay : Display
  FlowGain : Gain
  FlowSum : Sum  Inputs=2  SaturateOnIntegerOverflow=on  InputSameDT=on  OutDataTypeStr=Inherit: Same as first input
  Flow_PullO1BoxIIValveHydroNonStandard : Scope
      settings: Tag=Flow
  PotDisplay : Display
  Pot_PullO1BoxIIValveHydroNonStandard : Scope
      settings: Tag=Pot
  Rate Transition : RateTransition  OutPortSampleTimeMultiple=nT  OutPortSampleTime=Ts
  OutPot : Outport
  OutFlow : Outport  Tag=NOFLUX  Port=2
  wires:
  Rate Transition/1 -> OutPot/1
  InPot/1 -> Rate Transition/1, PotDisplay/1, Pot_PullO1BoxIIValveHydroNonStandard/1
  FlowGain/1 -> OutFlow/1, Flow_PullO1BoxIIValveHydroNonStandard/1, FlowDisplay/1
  FlowSum/1 -> FlowGain/1
  [PushO3BoxXValveHydroNonStandard] -> FlowSum/1
  [PushInertiaChamber1CylinderHydroNonStandard] -> FlowSum/2

== system Simple_lib/Hydraulic/Heat Sink/Linear Heat Pipe1/Push ==
  InPot : Inport
  InFlow : Inport  Tag=NOFLUX  Port=2
  FlowDisplay : Display
  Flow_PushO1BoxIIValveHydroNonStandard : Scope
      settings: Tag=Flow
  PotDisplay : Display
  Pot_PushO1BoxIIValveHydroNonStandard : Scope
      settings: Tag=Pot
  Rate Transition : RateTransition  OutPortSampleTimeMultiple=Ts  OutPortSampleTime=Ts
  OutPot : Outport  Tag=NOFLUX
  tag scope: PushO1BoxIIValveHydroNonStandard=global
  wires:
  Rate Transition/1 -> PotDisplay/1, Pot_PushO1BoxIIValveHydroNonStandard/1, OutPot/1
  InFlow/1 -> [PushO1BoxIIValveHydroNonStandard], FlowDisplay/1, Flow_PushO1BoxIIValveHydroNonStandard/1
  InPot/1 -> Rate Transition/1

== system Simple_lib/Hydraulic/Heat Sink/Linear Heat Pipe2/Pull ==
  InPot : Inport  Tag=NOFLUX
  FlowDisplay : Display
  FlowGain : Gain
  FlowSum : Sum  Inputs=2  SaturateOnIntegerOverflow=on  InputSameDT=on  OutDataTypeStr=Inherit: Same as first input
  Flow_PullO1BoxIIValveHydroNonStandard : Scope
      settings: Tag=Flow
  PotDisplay : Display
  Pot_PullO1BoxIIValveHydroNonStandard : Scope
      settings: Tag=Pot
  Rate Transition : RateTransition  OutPortSampleTimeMultiple=nT  OutPortSampleTime=Ts
  OutPot : Outport
  OutFlow : Outport  Tag=NOFLUX  Port=2
  wires:
  Rate Transition/1 -> OutPot/1
  InPot/1 -> Rate Transition/1, PotDisplay/1, Pot_PullO1BoxIIValveHydroNonStandard/1
  FlowGain/1 -> OutFlow/1, Flow_PullO1BoxIIValveHydroNonStandard/1, FlowDisplay/1
  FlowSum/1 -> FlowGain/1
  [PushO3BoxXValveHydroNonStandard] -> FlowSum/1
  [PushInertiaChamber1CylinderHydroNonStandard] -> FlowSum/2

== system Simple_lib/Hydraulic/Heat Sink/Linear Heat Pipe2/Push ==
  InPot : Inport
  InFlow : Inport  Tag=NOFLUX  Port=2
  FlowDisplay : Display
  Flow_PushO1BoxIIValveHydroNonStandard : Scope
      settings: Tag=Flow
  PotDisplay : Display
  Pot_PushO1BoxIIValveHydroNonStandard : Scope
      settings: Tag=Pot
  Rate Transition : RateTransition  OutPortSampleTimeMultiple=Ts  OutPortSampleTime=Ts
  OutPot : Outport  Tag=NOFLUX
  tag scope: PushO1BoxIIValveHydroNonStandard=global
  wires:
  Rate Transition/1 -> PotDisplay/1, Pot_PushO1BoxIIValveHydroNonStandard/1, OutPot/1
  InFlow/1 -> [PushO1BoxIIValveHydroNonStandard], FlowDisplay/1, Flow_PushO1BoxIIValveHydroNonStandard/1
  InPot/1 -> Rate Transition/1

== system Simple_lib/Hydraulic/Heat Sink/Linear Heat Pipe3/Pull ==
  InPot : Inport  Tag=NOFLUX
  FlowDisplay : Display
  FlowGain : Gain
  FlowSum : Sum  Inputs=2  SaturateOnIntegerOverflow=on  InputSameDT=on  OutDataTypeStr=Inherit: Same as first input
  Flow_PullO1BoxIIValveHydroNonStandard : Scope
      settings: Tag=Flow
  PotDisplay : Display
  Pot_PullO1BoxIIValveHydroNonStandard : Scope
      settings: Tag=Pot
  Rate Transition : RateTransition  OutPortSampleTimeMultiple=nT  OutPortSampleTime=Ts
  OutPot : Outport
  OutFlow : Outport  Tag=NOFLUX  Port=2
  wires:
  Rate Transition/1 -> OutPot/1
  InPot/1 -> Rate Transition/1, PotDisplay/1, Pot_PullO1BoxIIValveHydroNonStandard/1
  FlowGain/1 -> OutFlow/1, Flow_PullO1BoxIIValveHydroNonStandard/1, FlowDisplay/1
  FlowSum/1 -> FlowGain/1
  [PushO3BoxXValveHydroNonStandard] -> FlowSum/1
  [PushInertiaChamber1CylinderHydroNonStandard] -> FlowSum/2

== system Simple_lib/Hydraulic/Heat Sink/Linear Heat Pipe3/Push ==
  InPot : Inport
  InFlow : Inport  Tag=NOFLUX  Port=2
  FlowDisplay : Display
  Flow_PushO1BoxIIValveHydroNonStandard : Scope
      settings: Tag=Flow
  PotDisplay : Display
  Pot_PushO1BoxIIValveHydroNonStandard : Scope
      settings: Tag=Pot
  Rate Transition : RateTransition  OutPortSampleTimeMultiple=Ts  OutPortSampleTime=Ts
  OutPot : Outport  Tag=NOFLUX
  tag scope: PushO1BoxIIValveHydroNonStandard=global
  wires:
  Rate Transition/1 -> PotDisplay/1, Pot_PushO1BoxIIValveHydroNonStandard/1, OutPot/1
  InFlow/1 -> [PushO1BoxIIValveHydroNonStandard], FlowDisplay/1, Flow_PushO1BoxIIValveHydroNonStandard/1
  InPot/1 -> Rate Transition/1

== system Simple_lib/Hydraulic/Heat Sink/R1/Simplex ==
  InPot : Inport
  InFlow : Inport  Tag=NOFLUX  Port=2
  FlowDisplay : Display
  Flow_SimplexR17HeatExchangerFessSchematicSimulinkThermalFluid : Scope
      settings: Tag=Flow
  PotDisplay : Display
  Pot_SimplexR17HeatExchangerFessSchematicSimulinkThermalFluid : Scope
      settings: Tag=Pot
  Rate Transition : RateTransition  OutPortSampleTimeMultiple=Ts  OutPortSampleTime=Ts
  OutPot : Outport  Tag=NOFLUX
  tag scope: SimplexR17HeatExchangerFessSchematicSimulinkThermalFluid=global
  wires:
  InPot/1 -> Rate Transition/1
  InFlow/1 -> Flow_SimplexR17HeatExchangerFessSchematicSimulinkThermalFluid/1, FlowDisplay/1, [SimplexR17HeatExchangerFessSchematicSimulinkThermalFluid]
  Rate Transition/1 -> OutPot/1, Pot_SimplexR17HeatExchangerFessSchematicSimulinkThermalFluid/1, PotDisplay/1

== system Simple_lib/Hydraulic/Heat Sink/R1/Simplex1 ==
  InPot : Inport
  InFlow : Inport  Tag=NOFLUX  Port=2
  FlowDisplay : Display
  Flow_Simplex1R17HeatExchangerFessSchematicSimulinkThermalFluid : Scope
      settings: Tag=Flow
  PotDisplay : Display
  Pot_Simplex1R17HeatExchangerFessSchematicSimulinkThermalFluid : Scope
      settings: Tag=Pot
  Rate Transition : RateTransition  OutPortSampleTimeMultiple=Ts  OutPortSampleTime=Ts
  OutPot : Outport  Tag=NOFLUX
  tag scope: Simplex1R17HeatExchangerFessSchematicSimulinkThermalFluid=global
  wires:
  InPot/1 -> Rate Transition/1
  InFlow/1 -> Flow_Simplex1R17HeatExchangerFessSchematicSimulinkThermalFluid/1, FlowDisplay/1, [Simplex1R17HeatExchangerFessSchematicSimulinkThermalFluid]
  Rate Transition/1 -> OutPot/1, Pot_Simplex1R17HeatExchangerFessSchematicSimulinkThermalFluid/1, PotDisplay/1

== system Simple_lib/Hydraulic/Motor/Inertia/Duplex ==
  InPot : Inport  Tag=NOFLUX
  FlowDisplay : Display
  FlowGain : Gain
  FlowSum : Sum  Inputs=2  SaturateOnIntegerOverflow=on  InputSameDT=on  OutDataTypeStr=Inherit: Same as first input
  Flow_DuplexInertiaMotor2FessSchematicSimulink : Scope
      settings: Tag=Flow
  PotDisplay : Display
  Pot_DuplexInertiaMotor2FessSchematicSimulink : Scope
      settings: Tag=Pot
  Rate Transition : RateTransition  OutPortSampleTimeOpt=Multiple of input port sample time  OutPortSampleTimeMultiple=nT
  OutPot : Outport
  OutFlow : Outport  Tag=NOFLUX  Port=2
  wires:
  [PushBackMotor2FessSchematicSimulink] -> FlowSum/2
  [PushBack2VacuumPumpFessSchematicSimulink] -> FlowSum/1
  FlowSum/1 -> FlowGain/1
  FlowGain/1 -> FlowDisplay/1, Flow_DuplexInertiaMotor2FessSchematicSimulink/1, OutFlow/1
  InPot/1 -> Pot_DuplexInertiaMotor2FessSchematicSimulink/1, PotDisplay/1, Rate Transition/1
  Rate Transition/1 -> OutPot/1

== system Simple_lib/Hydraulic/Water-Glycol Heat Exchanger/Pipe1/Pull ==
  InPot : Inport  Tag=NOFLUX
  FlowDisplay : Display
  FlowGain : Gain
  Flow_PullPipe1WaterGlycolHeatExchangerFessSchematicSimulink : Scope
      settings: Tag=Flow
  PotDisplay : Display
  Pot_PullPipe1WaterGlycolHeatExchangerFessSchematicSimulink : Scope
      settings: Tag=Pot
  Rate Transition : RateTransition  OutPortSampleTimeMultiple=nT  OutPortSampleTime=Ts
  OutPot : Outport
  OutFlow : Outport  Tag=NOFLUX  Port=2
  wires:
  Rate Transition/1 -> OutPot/1
  InPot/1 -> Rate Transition/1, PotDisplay/1, Pot_PullPipe1WaterGlycolHeatExchangerFessSchematicSimulink/1
  FlowGain/1 -> OutFlow/1, Flow_PullPipe1WaterGlycolHeatExchangerFessSchematicSimulink/1, FlowDisplay/1

== system Simple_lib/Hydraulic/Water-Glycol Heat Exchanger/Pipe1/Push ==
  InPot : Inport
  InFlow : Inport  Tag=NOFLUX  Port=2
  FlowDisplay : Display
  Flow_PushPipe1WaterGlycolHeatExchangerFessSchematicSimulink : Scope
      settings: Tag=Flow
  PotDisplay : Display
  Pot_PushPipe1WaterGlycolHeatExchangerFessSchematicSimulink : Scope
      settings: Tag=Pot
  Rate Transition : RateTransition  OutPortSampleTimeMultiple=Ts  OutPortSampleTime=Ts
  OutPot : Outport  Tag=NOFLUX
  tag scope: PushPipe1WaterGlycolHeatExchangerFessSchematicSimulink=global
  wires:
  Rate Transition/1 -> PotDisplay/1, Pot_PushPipe1WaterGlycolHeatExchangerFessSchematicSimulink/1, OutPot/1
  InFlow/1 -> [PushPipe1WaterGlycolHeatExchangerFessSchematicSimulink], FlowDisplay/1, Flow_PushPipe1WaterGlycolHeatExchangerFessSchematicSimulink/1
  InPot/1 -> Rate Transition/1

== system Simple_lib/Hydraulic/Water-Glycol Heat Exchanger/Pipe2/Pull ==
  InPot : Inport  Tag=NOFLUX
  FlowDisplay : Display
  FlowGain : Gain
  Flow_PullPipe2WaterGlycolHeatExchangerFessSchematicSimulink : Scope
      settings: Tag=Flow
  PotDisplay : Display
  Pot_PullPipe2WaterGlycolHeatExchangerFessSchematicSimulink : Scope
      settings: Tag=Pot
  Rate Transition : RateTransition  OutPortSampleTimeMultiple=nT  OutPortSampleTime=Ts
  OutPot : Outport
  OutFlow : Outport  Tag=NOFLUX  Port=2
  wires:
  Rate Transition/1 -> OutPot/1
  InPot/1 -> Rate Transition/1, PotDisplay/1, Pot_PullPipe2WaterGlycolHeatExchangerFessSchematicSimulink/1
  FlowGain/1 -> OutFlow/1, Flow_PullPipe2WaterGlycolHeatExchangerFessSchematicSimulink/1, FlowDisplay/1

== system Simple_lib/Hydraulic/Water-Glycol Heat Exchanger/Pipe2/Push ==
  InPot : Inport
  InFlow : Inport  Tag=NOFLUX  Port=2
  FlowDisplay : Display
  Flow_PushPipe2WaterGlycolHeatExchangerFessSchematicSimulink : Scope
      settings: Tag=Flow
  PotDisplay : Display
  Pot_PushPipe2WaterGlycolHeatExchangerFessSchematicSimulink : Scope
      settings: Tag=Pot
  Rate Transition : RateTransition  OutPortSampleTimeMultiple=Ts  OutPortSampleTime=Ts
  OutPot : Outport  Tag=NOFLUX
  tag scope: PushPipe2WaterGlycolHeatExchangerFessSchematicSimulink=global
  wires:
  Rate Transition/1 -> PotDisplay/1, Pot_PushPipe2WaterGlycolHeatExchangerFessSchematicSimulink/1, OutPot/1
  InFlow/1 -> [PushPipe2WaterGlycolHeatExchangerFessSchematicSimulink], FlowDisplay/1, Flow_PushPipe2WaterGlycolHeatExchangerFessSchematicSimulink/1
  InPot/1 -> Rate Transition/1
